simulink model "Cooperative_Quad_09_VelEst_02"  (R2017b)
settings: Solver=ode45  StartTime=0.0  StopTime=120  RelTol=1e-3  EnableMultiTasking=on
InitFcn:
  | Const_Vel_Est_02
values from neighbouring files (symbols this model uses):
  alpha = 1.0e-5    (= 1e-05)    [Cons_AMFC_Quad_New_01.m]    (also in Const_Vel_Est_02.m = 0.1; constant_Rev01_4Agents_10.m = 0.1; constant_Rev01_4Agents_9.m = 0.1)
  alpha_Slid = 0.01    [Cons_AMFC_Quad_New_01.m]    (also in Const_Vel_Est_02.m)
  AN = [     0 1 0 0 ... (first row only)    [Const_Vel_Est_02.m]    (also in constant_Rev01_4Agents_10.m; constant_Rev01_4Agents_9.m)
  B = 1e+0*eye(n)    [Cons_AMFC_Quad_New_01.m]    (also in Const_Vel_Est_02.m = 1e0*eye(n); constant_Rev01_4Agents_10.m = 1e0*eye(n); constant_Rev01_4Agents_9.m = 1e0*eye(n))
  BBT_inv = ((B'*B)^(-1))*B'    [Cons_AMFC_Quad_New_01.m]    (also in Const_Vel_Est_02.m; constant_Rev01_4Agents_10.m; constant_Rev01_4Agents_9.m)
  BN = [     1 0 0 0 ... (first row only)    [Const_Vel_Est_02.m]    (also in constant_Rev01_4Agents_10.m; constant_Rev01_4Agents_9.m)
  epsilon_struct = struct('data',epsilon_InitVal)    [Const_Vel_Est_02.m]    (also in constant_Rev01_4Agents_10.m; constant_Rev01_4Agents_9.m)
  g = 9.81    [Const_Vel_Est_02.m]    (also in Swing2d_01_const.m; constant_Rev01_4Agents_10.m; constant_Rev01_4Agents_9.m)
  gamma_0 = 1e-0*diag([1e-3*ones(3,1);1e-0*ones(3,1)])    [Cons_AMFC_Quad_New_01.m]    (also in Const_Vel_Est_02.m = 1e-1*diag([1e-3*ones(3,1);1e-0*ones(3,1)]); constant_Rev01_4Agents_10.m = 1e+1*diag([1e-3*ones(3,1);1e-0*ones(3,1)]); constant_Rev01_4Agents_9.m = 1e+1*diag([1e-3*ones(6,1);1e-0*ones(6,1)]))
  gamma_1 = 1e+2*diag([1e-3*ones(3,1);1e-0*ones(3,1)])    [Cons_AMFC_Quad_New_01.m]    (also in Const_Vel_Est_02.m; constant_Rev01_4Agents_10.m = 1e+3*diag([1e-3*ones(3,1);1e0*ones(3,1)]); constant_Rev01_4Agents_9.m = 1e+3*diag([1e-3*ones(6,1);1e0*ones(6,1)]))
  H = L + BN    [Const_Vel_Est_02.m]    (also in constant_Rev01_4Agents_10.m; constant_Rev01_4Agents_9.m)
  J = 1.2416e-3 * diag([1 1 2])    [Cons_AMFC_Quad_New_01.m]    (also in Const_Vel_Est_02.m = 1.2416e-3 * diag([1 1 2],0); constant_Rev01_4Agents_10.m = 1.2416e-3 * diag([1 1 2],0); constant_Rev01_4Agents_9.m = 1.2416e-3 * diag([1 1 2],0))
  k1 = 10    [Cons_AMFC_Quad_New_01.m]    (also in Const_Vel_Est_02.m = 1; constant_Rev01_4Agents_10.m = 1; constant_Rev01_4Agents_9.m = 1)
  k1o = 1000    [Cons_AMFC_Quad_New_01.m]    (also in Const_Vel_Est_02.m)
  k2 = 0.1    [Cons_AMFC_Quad_New_01.m]    (also in Const_Vel_Est_02.m; constant_Rev01_4Agents_10.m = 1; constant_Rev01_4Agents_9.m = 1)
  k2o = 100    [Cons_AMFC_Quad_New_01.m]    (also in Const_Vel_Est_02.m)
  Ka = 0.01    [Cons_AMFC_Quad_New_01.m]    (also in Const_Vel_Est_02.m; constant_Rev01_4Agents_10.m; constant_Rev01_4Agents_9.m)
  Kd = 0.01    [Cons_AMFC_Quad_New_01.m]    (also in Const_Vel_Est_02.m; constant_Rev01_4Agents_10.m; constant_Rev01_4Agents_9.m)
  Kf = 1.0e-5    (= 1e-05)    [Cons_AMFC_Quad_New_01.m]    (also in Const_Vel_Est_02.m; constant_Rev01_4Agents_10.m; constant_Rev01_4Agents_9.m)
  Kt = 0.0435 * Kf    (= 4.35e-07)    [Cons_AMFC_Quad_New_01.m]    (also in Const_Vel_Est_02.m = 1e-07; constant_Rev01_4Agents_10.m = 1e-07; constant_Rev01_4Agents_9.m = 1e-07)
  Lq = 0.2    [Const_Vel_Est_02.m]    (also in constant_Rev01_4Agents_10.m; constant_Rev01_4Agents_9.m)
  m = 6    [Cons_AMFC_Quad_New_01.m]    (also in Const_Vel_Est_02.m; Swing2d_01_const.m = 1)
  M = 2.95    [Cons_AMFC_Quad_New_01.m]    (also in Const_Vel_Est_02.m = 2; constant_Rev01_4Agents_10.m = 2; constant_Rev01_4Agents_9.m = 2)
  Mb_P = Mb_val_P*ones(np,1)    [Const_Vel_Est_02.m]
  Mb_V = Mb_val_V*ones(np,1)    [Const_Vel_Est_02.m]
  Mu_P = 10    [Const_Vel_Est_02.m]
  Mu_V = 10    [Const_Vel_Est_02.m]
  n = 6    [Cons_AMFC_Quad_New_01.m]    (also in Const_Vel_Est_02.m; constant_Rev01_4Agents_10.m; constant_Rev01_4Agents_9.m = 12)
  N = 4    [Const_Vel_Est_02.m]    (also in constant_Rev01_4Agents_10.m; constant_Rev01_4Agents_9.m)
  n0 = 3    [Const_Vel_Est_02.m]    (also in constant_Rev01_4Agents_10.m; constant_Rev01_4Agents_9.m)
  np = 2    [Const_Vel_Est_02.m]
  Observer_Gain = 100    [Const_Vel_Est_02.m]    (also in constant_Rev01_4Agents_10.m; constant_Rev01_4Agents_9.m)
  Observer_Gain1 = 100    [Const_Vel_Est_02.m]    (also in constant_Rev01_4Agents_10.m = 10; constant_Rev01_4Agents_9.m = 10)
  Q = 1e-1*eye(n)    [Cons_AMFC_Quad_New_01.m]    (also in Const_Vel_Est_02.m = 1e-2*eye(n); constant_Rev01_4Agents_10.m = 1e-3*eye(n); constant_Rev01_4Agents_9.m = 1e-3*eye(n))
  R = 1e+0*eye(m)    [Cons_AMFC_Quad_New_01.m]    (also in Const_Vel_Est_02.m = 1e-0*eye(n); constant_Rev01_4Agents_10.m = 1e-0*eye(n); constant_Rev01_4Agents_9.m = 1e-0*eye(n))
  rho_0 = 1e-1    (= 0.1)    [Cons_AMFC_Quad_New_01.m]    (also in Const_Vel_Est_02.m; constant_Rev01_4Agents_10.m = 10; constant_Rev01_4Agents_9.m = 10)
  rho_1 = 1e-0    (= 1)    [Cons_AMFC_Quad_New_01.m]    (also in Const_Vel_Est_02.m; constant_Rev01_4Agents_10.m = 0.1; constant_Rev01_4Agents_9.m = 0.1)
  T_struct = struct('data',T_InitVal)    [Const_Vel_Est_02.m]    (also in constant_Rev01_4Agents_10.m; constant_Rev01_4Agents_9.m)
  U_dot0_M = U_dot0_m*ones(n0,1)    [Const_Vel_Est_02.m]    (also in constant_Rev01_4Agents_10.m; constant_Rev01_4Agents_9.m)
  Upsilon_M = Upsilon_m*ones(n0,1)    [Const_Vel_Est_02.m]    (also in constant_Rev01_4Agents_10.m; constant_Rev01_4Agents_9.m)
undefined symbols (not defined in the file or in its folder): sigbuilder_block
(part 3 of 5)

== system Cooperative_Quad_09_VelEst_02/Agent #2/Relative estimations-2/Rel_24/Differentiator1 ==
  x_d : Inport
  Constant : Constant  Value=zeros(3,1)
  Gain : Gain
  Integrator : Integrator
  Integrator1 : Integrator
  Sliding differentiator : MATLAB Function  TreatAsAtomicUnit=on
  Sliding differentiator1 : MATLAB Function  TreatAsAtomicUnit=on
  Sum : Sum  Inputs=|-+
  Dx_d : Outport
  wires:
  Sliding differentiator/1(u) -> Integrator1/1, Dx_d/1
  Gain/1 -> Sum/2
  Integrator1/1 -> Gain/1
  Sum/1 -> Sliding differentiator1/1(e), Sliding differentiator/2(e)
  x_d/1 -> Sum/1
  Integrator/1 -> Sliding differentiator/1(u1)
  Sliding differentiator1/1(Du1) -> Integrator/1

== system Cooperative_Quad_09_VelEst_02/Agent #3/Decenteralized Cooperaive Controller #3/Ali-3/Rotational-3 ==
  x_rd : Inport
  X : Inport  Port=2
  CARE : MATLAB Function  TreatAsAtomicUnit=on
  Differentiator : Subsystem
  Integrator : Integrator  InitialCondition=zeros(n)
  Integrator1 : Integrator  InitialCondition=eye(n)
  Integrator2 : Integrator  InitialCondition=zeros(n,1)
  Integrator3 : Integrator  InitialCondition=zeros(n,1)
  Memory : Memory  InitialCondition=zeros(m,1)
  Sum : Sum  Inputs=|++
  g-Estimator : MATLAB Function  TreatAsAtomicUnit=on
  g-Estimator1 : MATLAB Function  TreatAsAtomicUnit=on
  main : MATLAB Function  TreatAsAtomicUnit=on
  variable change : MATLAB Function  TreatAsAtomicUnit=on
  ur : Outport
  tag scope: A_hat3_R=global, P3_R=global, g_hat3_R=global, u3_R=global
  wires:
  x_rd/1 -> variable change/2(Xd)
  X/1 -> variable change/1(X)
  CARE/1(DP) -> Integrator1/1
  Sum/1 -> main/1(sigma), g-Estimator/1(sigma), g-Estimator1/1(sigma)
  g-Estimator1/1(Da_hat) -> Integrator/1
  variable change/1(x_mod) -> main/7(x), g-Estimator1/2(x)
  Integrator1/1 -> [P3_R], g-Estimator1/3(P), CARE/1(P), g-Estimator/3(P), main/4(P)
  Integrator/1 -> g-Estimator1/4(a_hat), CARE/2(a_hat), [A_hat3_R], main/5(a_hat)
  g-Estimator/1(Dg_hat) -> Integrator2/1
  Differentiator/1(Dx_d) -> main/3(Dy_d)
  main/1(u) -> [u3_R], Memory/1, ur/1
  Integrator3/1 -> main/2(zeta), Sum/1
  variable change/2(xd_mod) -> Differentiator/1(x_d)
  variable change/3(e_mod) -> Sum/2, Integrator3/1
  Memory/1 -> variable change/3(u)
  Integrator2/1 -> g-Estimator/2(g_hat), [g_hat3_R], main/6(g_hat)

== system Cooperative_Quad_09_VelEst_02/Agent #3/Decenteralized Cooperaive Controller #3/Ali-3/Translational-3 ==
  x_td : Inport
  x_t : Inport  Port=2
  A-Estimator : MATLAB Function  TreatAsAtomicUnit=on
  CARE : MATLAB Function  TreatAsAtomicUnit=on
  Differentiator : Subsystem
  Integrator : Integrator  InitialCondition=zeros(n)
  Integrator1 : Integrator  InitialCondition=eye(n)
  Integrator2 : Integrator  InitialCondition=zeros(n,1)
  Integrator3 : Integrator  InitialCondition=zeros(n,1)
  Memory : Memory  InitialCondition=zeros(m,1)
  Sum : Sum  Inputs=|++
  g-Estimator : MATLAB Function  TreatAsAtomicUnit=on
  main : MATLAB Function  TreatAsAtomicUnit=on
  variable change : MATLAB Function  TreatAsAtomicUnit=on
  ut : Outport
  tag scope: A_hat3_T=global, P3_T=global, g_hat3_T=global, u3_T=global
  wires:
  Integrator2/1 -> [g_hat3_T], main/6(g_hat), g-Estimator/2(g_hat)
  Memory/1 -> variable change/3(u)
  variable change/3(e_mod) -> Integrator3/1, Sum/2
  variable change/2(xd_mod) -> Differentiator/1(x_d)
  Integrator3/1 -> Sum/1, main/2(zeta)
  main/1(u) -> ut/1, [u3_T], Memory/1
  Differentiator/1(Dx_d) -> main/3(Dy_d)
  g-Estimator/1(Dg_hat) -> Integrator2/1
  Integrator/1 -> [A_hat3_T], main/5(a_hat), CARE/2(a_hat), A-Estimator/4(a_hat)
  Integrator1/1 -> main/4(P), g-Estimator/3(P), CARE/1(P), [P3_T], A-Estimator/3(P)
  variable change/1(x_mod) -> A-Estimator/2(x), main/7(x)
  A-Estimator/1(Da_hat) -> Integrator/1
  Sum/1 -> A-Estimator/1(sigma), g-Estimator/1(sigma), main/1(sigma)
  CARE/1(DP) -> Integrator1/1
  x_td/1 -> variable change/2(Xd)
  x_t/1 -> variable change/1(X)

== system Cooperative_Quad_09_VelEst_02/Agent #3/Decenteralized Cooperaive Controller #3/Cooperative Observers for X-3/Differentiator2 ==
  Pos_Z : Inport
  Integrator : Integrator
  Integrator1 : Integrator
  Sliding differentiator : MATLAB Function  TreatAsAtomicUnit=on
  Sliding differentiator1 : MATLAB Function  TreatAsAtomicUnit=on
  Sum : Sum  Inputs=|-+
  DPos_Z : Outport
  wires:
  Sliding differentiator/1(u) -> Integrator1/1, DPos_Z/1
  Integrator1/1 -> Sum/2
  Sum/1 -> Sliding differentiator1/1(e), Sliding differentiator/2(e)
  Pos_Z/1 -> Sum/1
  Integrator/1 -> Sliding differentiator/1(u1)
  Sliding differentiator1/1(Du1) -> Integrator/1

== system Cooperative_Quad_09_VelEst_02/Agent #3/Relative estimations-3/Rel_30/Differentiator1 ==
  x_d : Inport
  Constant : Constant  Value=zeros(3,1)
  Gain : Gain
  Integrator : Integrator
  Integrator1 : Integrator
  Sliding differentiator : MATLAB Function  TreatAsAtomicUnit=on
  Sliding differentiator1 : MATLAB Function  TreatAsAtomicUnit=on
  Sum : Sum  Inputs=|-+
  Dx_d : Outport
  wires:
  Sliding differentiator/1(u) -> Integrator1/1, Dx_d/1
  Gain/1 -> Sum/2
  Integrator1/1 -> Gain/1
  Sum/1 -> Sliding differentiator1/1(e), Sliding differentiator/2(e)
  x_d/1 -> Sum/1
  Integrator/1 -> Sliding differentiator/1(u1)
  Sliding differentiator1/1(Du1) -> Integrator/1

== system Cooperative_Quad_09_VelEst_02/Agent #3/Relative estimations-3/Rel_31/Differentiator1 ==
  x_d : Inport
  Constant : Constant  Value=zeros(3,1)
  Gain : Gain
  Integrator : Integrator
  Integrator1 : Integrator
  Sliding differentiator : MATLAB Function  TreatAsAtomicUnit=on
  Sliding differentiator1 : MATLAB Function  TreatAsAtomicUnit=on
  Sum : Sum  Inputs=|-+
  Dx_d : Outport
  wires:
  Sliding differentiator1/1(Du1) -> Integrator/1
  Integrator/1 -> Sliding differentiator/1(u1)
  x_d/1 -> Sum/1
  Sum/1 -> Sliding differentiator/2(e), Sliding differentiator1/1(e)
  Integrator1/1 -> Gain/1
  Gain/1 -> Sum/2
  Sliding differentiator/1(u) -> Dx_d/1, Integrator1/1

== system Cooperative_Quad_09_VelEst_02/Agent #3/Relative estimations-3/Rel_32/Differentiator1 ==
  x_d : Inport
  Constant : Constant  Value=zeros(3,1)
  Gain : Gain
  Integrator : Integrator
  Integrator1 : Integrator
  Sliding differentiator : MATLAB Function  TreatAsAtomicUnit=on
  Sliding differentiator1 : MATLAB Function  TreatAsAtomicUnit=on
  Sum : Sum  Inputs=|-+
  Dx_d : Outport
  wires:
  Sliding differentiator/1(u) -> Integrator1/1, Dx_d/1
  Gain/1 -> Sum/2
  Integrator1/1 -> Gain/1
  Sum/1 -> Sliding differentiator1/1(e), Sliding differentiator/2(e)
  x_d/1 -> Sum/1
  Integrator/1 -> Sliding differentiator/1(u1)
  Sliding differentiator1/1(Du1) -> Integrator/1

== system Cooperative_Quad_09_VelEst_02/Agent #3/Relative estimations-3/Rel_34/Differentiator1 ==
  x_d : Inport
  Constant : Constant  Value=zeros(3,1)
  Gain : Gain
  Integrator : Integrator
  Integrator1 : Integrator
  Sliding differentiator : MATLAB Function  TreatAsAtomicUnit=on
  Sliding differentiator1 : MATLAB Function  TreatAsAtomicUnit=on
  Sum : Sum  Inputs=|-+
  Dx_d : Outport
  wires:
  Sliding differentiator1/1(Du1) -> Integrator/1
  Integrator/1 -> Sliding differentiator/1(u1)
  x_d/1 -> Sum/1
  Sum/1 -> Sliding differentiator/2(e), Sliding differentiator1/1(e)
  Integrator1/1 -> Gain/1
  Gain/1 -> Sum/2
  Sliding differentiator/1(u) -> Dx_d/1, Integrator1/1

== system Cooperative_Quad_09_VelEst_02/Agent #4/Decenteralized Cooperaive Controller #4/Ali-4/Rotational-4 ==
  x_rd : Inport
  X : Inport  Port=2
  CARE : MATLAB Function  TreatAsAtomicUnit=on
  Differentiator : Subsystem
  Integrator : Integrator  InitialCondition=zeros(n)
  Integrator1 : Integrator  InitialCondition=eye(n)
  Integrator2 : Integrator  InitialCondition=zeros(n,1)
  Integrator3 : Integrator  InitialCondition=zeros(n,1)
  Memory : Memory  InitialCondition=zeros(m,1)
  Sum : Sum  Inputs=|++
  g-Estimator : MATLAB Function  TreatAsAtomicUnit=on
  g-Estimator1 : MATLAB Function  TreatAsAtomicUnit=on
  main : MATLAB Function  TreatAsAtomicUnit=on
  variable change : MATLAB Function  TreatAsAtomicUnit=on
  ur : Outport
  tag scope: A_hat4_R=global, P4_R=global, g_hat4_R=global, u4_R=global
  wires:
  Integrator2/1 -> main/6(g_hat), [g_hat4_R], g-Estimator/2(g_hat)
  Memory/1 -> variable change/3(u)
  variable change/3(e_mod) -> Integrator3/1, Sum/2
  variable change/2(xd_mod) -> Differentiator/1(x_d)
  Integrator3/1 -> Sum/1, main/2(zeta)
  main/1(u) -> ur/1, Memory/1, [u4_R]
  Differentiator/1(Dx_d) -> main/3(Dy_d)
  g-Estimator/1(Dg_hat) -> Integrator2/1
  Integrator/1 -> main/5(a_hat), [A_hat4_R], CARE/2(a_hat), g-Estimator1/4(a_hat)
  Integrator1/1 -> main/4(P), g-Estimator/3(P), CARE/1(P), g-Estimator1/3(P), [P4_R]
  variable change/1(x_mod) -> g-Estimator1/2(x), main/7(x)
  g-Estimator1/1(Da_hat) -> Integrator/1
  Sum/1 -> g-Estimator1/1(sigma), g-Estimator/1(sigma), main/1(sigma)
  CARE/1(DP) -> Integrator1/1
  X/1 -> variable change/1(X)
  x_rd/1 -> variable change/2(Xd)

== system Cooperative_Quad_09_VelEst_02/Agent #4/Decenteralized Cooperaive Controller #4/Ali-4/Translational-4 ==
  x_td : Inport
  x_t : Inport  Port=2
  A-Estimator : MATLAB Function  TreatAsAtomicUnit=on
  CARE : MATLAB Function  TreatAsAtomicUnit=on
  Differentiator : Subsystem
  Integrator : Integrator  InitialCondition=zeros(n)
  Integrator1 : Integrator  InitialCondition=eye(n)
  Integrator2 : Integrator  InitialCondition=zeros(n,1)
  Integrator3 : Integrator  InitialCondition=zeros(n,1)
  Memory : Memory  InitialCondition=zeros(m,1)
  Sum : Sum  Inputs=|++
  g-Estimator : MATLAB Function  TreatAsAtomicUnit=on
  main : MATLAB Function  TreatAsAtomicUnit=on
  variable change : MATLAB Function  TreatAsAtomicUnit=on
  ut : Outport
  tag scope: A_hat4_T=global, P4_T=global, g_hat4_T=global, u4_T=global
  wires:
  x_t/1 -> variable change/1(X)
  x_td/1 -> variable change/2(Xd)
  CARE/1(DP) -> Integrator1/1
  Sum/1 -> main/1(sigma), g-Estimator/1(sigma), A-Estimator/1(sigma)
  A-Estimator/1(Da_hat) -> Integrator/1
  variable change/1(x_mod) -> main/7(x), A-Estimator/2(x)
  Integrator1/1 -> A-Estimator/3(P), [P4_T], CARE/1(P), g-Estimator/3(P), main/4(P)
  Integrator/1 -> A-Estimator/4(a_hat), CARE/2(a_hat), main/5(a_hat), [A_hat4_T]
  g-Estimator/1(Dg_hat) -> Integrator2/1
  Differentiator/1(Dx_d) -> main/3(Dy_d)
  main/1(u) -> Memory/1, [u4_T], ut/1
  Integrator3/1 -> main/2(zeta), Sum/1
  variable change/2(xd_mod) -> Differentiator/1(x_d)
  variable change/3(e_mod) -> Sum/2, Integrator3/1
  Memory/1 -> variable change/3(u)
  Integrator2/1 -> g-Estimator/2(g_hat), main/6(g_hat), [g_hat4_T]

== system Cooperative_Quad_09_VelEst_02/Agent #4/Decenteralized Cooperaive Controller #4/Cooperative Observers for X-4/Differentiator2 ==
  Pos_Z : Inport
  Integrator : Integrator
  Integrator1 : Integrator
  Sliding differentiator : MATLAB Function  TreatAsAtomicUnit=on
  Sliding differentiator1 : MATLAB Function  TreatAsAtomicUnit=on
  Sum : Sum  Inputs=|-+
  DPos_Z : Outport
  wires:
  Sliding differentiator1/1(Du1) -> Integrator/1
  Integrator/1 -> Sliding differentiator/1(u1)
  Pos_Z/1 -> Sum/1
  Sum/1 -> Sliding differentiator/2(e), Sliding differentiator1/1(e)
  Integrator1/1 -> Sum/2
  Sliding differentiator/1(u) -> DPos_Z/1, Integrator1/1

== system Cooperative_Quad_09_VelEst_02/Agent #4/Relative estimations-4/Rel_40/Differentiator1 ==
  x_d : Inport
  Constant : Constant  Value=zeros(3,1)
  Gain : Gain
  Integrator : Integrator
  Integrator1 : Integrator
  Sliding differentiator : MATLAB Function  TreatAsAtomicUnit=on
  Sliding differentiator1 : MATLAB Function  TreatAsAtomicUnit=on
  Sum : Sum  Inputs=|-+
  Dx_d : Outport
  wires:
  Sliding differentiator1/1(Du1) -> Integrator/1
  Integrator/1 -> Sliding differentiator/1(u1)
  x_d/1 -> Sum/1
  Sum/1 -> Sliding differentiator/2(e), Sliding differentiator1/1(e)
  Integrator1/1 -> Gain/1
  Gain/1 -> Sum/2
  Sliding differentiator/1(u) -> Dx_d/1, Integrator1/1

== system Cooperative_Quad_09_VelEst_02/Agent #4/Relative estimations-4/Rel_41/Differentiator1 ==
  x_d : Inport
  Constant : Constant  Value=zeros(3,1)
  Gain : Gain
  Integrator : Integrator
  Integrator1 : Integrator
  Sliding differentiator : MATLAB Function  TreatAsAtomicUnit=on
  Sliding differentiator1 : MATLAB Function  TreatAsAtomicUnit=on
  Sum : Sum  Inputs=|-+
  Dx_d : Outport
  wires:
  Sliding differentiator/1(u) -> Integrator1/1, Dx_d/1
  Gain/1 -> Sum/2
  Integrator1/1 -> Gain/1
  Sum/1 -> Sliding differentiator1/1(e), Sliding differentiator/2(e)
  x_d/1 -> Sum/1
  Integrator/1 -> Sliding differentiator/1(u1)
  Sliding differentiator1/1(Du1) -> Integrator/1

== system Cooperative_Quad_09_VelEst_02/Agent #4/Relative estimations-4/Rel_42/Differentiator1 ==
  x_d : Inport
  Constant : Constant  Value=zeros(3,1)
  Gain : Gain
  Integrator : Integrator
  Integrator1 : Integrator
  Sliding differentiator : MATLAB Function  TreatAsAtomicUnit=on
  Sliding differentiator1 : MATLAB Function  TreatAsAtomicUnit=on
  Sum : Sum  Inputs=|-+
  Dx_d : Outport
  wires:
  Sliding differentiator1/1(Du1) -> Integrator/1
  Integrator/1 -> Sliding differentiator/1(u1)
  x_d/1 -> Sum/1
  Sum/1 -> Sliding differentiator/2(e), Sliding differentiator1/1(e)
  Integrator1/1 -> Gain/1
  Gain/1 -> Sum/2
  Sliding differentiator/1(u) -> Dx_d/1, Integrator1/1

== system Cooperative_Quad_09_VelEst_02/Agent #4/Relative estimations-4/Rel_43/Differentiator1 ==
  x_d : Inport
  Constant : Constant  Value=zeros(3,1)
  Gain : Gain
  Integrator : Integrator
  Integrator1 : Integrator
  Sliding differentiator : MATLAB Function  TreatAsAtomicUnit=on
  Sliding differentiator1 : MATLAB Function  TreatAsAtomicUnit=on
  Sum : Sum  Inputs=|-+
  Dx_d : Outport
  wires:
  Sliding differentiator/1(u) -> Integrator1/1, Dx_d/1
  Gain/1 -> Sum/2
  Integrator1/1 -> Gain/1
  Sum/1 -> Sliding differentiator1/1(e), Sliding differentiator/2(e)
  x_d/1 -> Sum/1
  Integrator/1 -> Sliding differentiator/1(u1)
  Sliding differentiator1/1(Du1) -> Integrator/1

== system Cooperative_Quad_09_VelEst_02/Agent #1/Decenteralized Cooperaive Controller #1/Ali-1/Rotational-1/Differentiator ==
  x_d : Inport
  Integrator : Integrator  InitialCondition=zeros(n,1)
  Integrator1 : Integrator  InitialCondition=zeros(n,1)
  Sliding differentiator : MATLAB Function  TreatAsAtomicUnit=on
  Sliding differentiator1 : MATLAB Function  TreatAsAtomicUnit=on
  Sum : Sum  Inputs=|-+
  Dx_d : Outport
  wires:
  Sliding differentiator/1(u) -> Integrator1/1, Dx_d/1
  Sliding differentiator1/1(Du1) -> Integrator/1
  Integrator/1 -> Sliding differentiator/1(u1)
  x_d/1 -> Sum/1
  Sum/1 -> Sliding differentiator/2(e), Sliding differentiator1/1(e)
  Integrator1/1 -> Sum/2

== system Cooperative_Quad_09_VelEst_02/Agent #1/Decenteralized Cooperaive Controller #1/Ali-1/Translational-1/Differentiator ==
  x_d : Inport
  Integrator : Integrator  InitialCondition=zeros(n,1)
  Integrator1 : Integrator  InitialCondition=zeros(n,1)
  Scope : Scope
  Scope1 : Scope
  Sliding differentiator : MATLAB Function  TreatAsAtomicUnit=on
  Sliding differentiator1 : MATLAB Function  TreatAsAtomicUnit=on
  Sum : Sum  Inputs=|-+
  Dx_d : Outport
  wires:
  Integrator1/1 -> Sum/2
  Sum/1 -> Sliding differentiator1/1(e), Sliding differentiator/2(e), Scope1/1
  x_d/1 -> Sum/1
  Integrator/1 -> Sliding differentiator/1(u1)
  Sliding differentiator1/1(Du1) -> Integrator/1
  Sliding differentiator/1(u) -> Dx_d/1, Integrator1/1, Scope/1

== system Cooperative_Quad_09_VelEst_02/Agent #2/Decenteralized Cooperaive Controller #2/Ali-2/Rotational-2/Differentiator ==
  x_d : Inport
  Integrator : Integrator  InitialCondition=zeros(n,1)
  Integrator1 : Integrator  InitialCondition=zeros(n,1)
  Sliding differentiator : MATLAB Function  TreatAsAtomicUnit=on
  Sliding differentiator1 : MATLAB Function  TreatAsAtomicUnit=on
  Sum : Sum  Inputs=|-+
  Dx_d : Outport
  wires:
  Integrator1/1 -> Sum/2
  Sum/1 -> Sliding differentiator1/1(e), Sliding differentiator/2(e)
  x_d/1 -> Sum/1
  Integrator/1 -> Sliding differentiator/1(u1)
  Sliding differentiator1/1(Du1) -> Integrator/1
  Sliding differentiator/1(u) -> Dx_d/1, Integrator1/1

== system Cooperative_Quad_09_VelEst_02/Agent #2/Decenteralized Cooperaive Controller #2/Ali-2/Translational-2/Differentiator ==
  x_d : Inport
  Integrator : Integrator  InitialCondition=zeros(n,1)
  Integrator1 : Integrator  InitialCondition=zeros(n,1)
  Scope : Scope
  Scope1 : Scope
  Sliding differentiator : MATLAB Function  TreatAsAtomicUnit=on
  Sliding differentiator1 : MATLAB Function  TreatAsAtomicUnit=on
  Sum : Sum  Inputs=|-+
  Dx_d : Outport
  wires:
  Sliding differentiator/1(u) -> Scope/1, Integrator1/1, Dx_d/1
  Sliding differentiator1/1(Du1) -> Integrator/1
  Integrator/1 -> Sliding differentiator/1(u1)
  x_d/1 -> Sum/1
  Sum/1 -> Scope1/1, Sliding differentiator/2(e), Sliding differentiator1/1(e)
  Integrator1/1 -> Sum/2

== system Cooperative_Quad_09_VelEst_02/Agent #3/Decenteralized Cooperaive Controller #3/Ali-3/Rotational-3/Differentiator ==
  x_d : Inport
  Integrator : Integrator  InitialCondition=zeros(n,1)
  Integrator1 : Integrator  InitialCondition=zeros(n,1)
  Sliding differentiator : MATLAB Function  TreatAsAtomicUnit=on
  Sliding differentiator1 : MATLAB Function  TreatAsAtomicUnit=on
  Sum : Sum  Inputs=|-+
  Dx_d : Outport
  wires:
  Sliding differentiator/1(u) -> Integrator1/1, Dx_d/1
  Sliding differentiator1/1(Du1) -> Integrator/1
  Integrator/1 -> Sliding differentiator/1(u1)
  x_d/1 -> Sum/1
  Sum/1 -> Sliding differentiator/2(e), Sliding differentiator1/1(e)
  Integrator1/1 -> Sum/2

== system Cooperative_Quad_09_VelEst_02/Agent #3/Decenteralized Cooperaive Controller #3/Ali-3/Translational-3/Differentiator ==
  x_d : Inport
  Integrator : Integrator  InitialCondition=zeros(n,1)
  Integrator1 : Integrator  InitialCondition=zeros(n,1)
  Scope : Scope
  Scope1 : Scope
  Sliding differentiator : MATLAB Function  TreatAsAtomicUnit=on
  Sliding differentiator1 : MATLAB Function  TreatAsAtomicUnit=on
  Sum : Sum  Inputs=|-+
  Dx_d : Outport
  wires:
  Integrator1/1 -> Sum/2
  Sum/1 -> Sliding differentiator1/1(e), Sliding differentiator/2(e), Scope1/1
  x_d/1 -> Sum/1
  Integrator/1 -> Sliding differentiator/1(u1)
  Sliding differentiator1/1(Du1) -> Integrator/1
  Sliding differentiator/1(u) -> Dx_d/1, Integrator1/1, Scope/1

== system Cooperative_Quad_09_VelEst_02/Agent #4/Decenteralized Cooperaive Controller #4/Ali-4/Rotational-4/Differentiator ==
  x_d : Inport
  Integrator : Integrator  InitialCondition=zeros(n,1)
  Integrator1 : Integrator  InitialCondition=zeros(n,1)
  Sliding differentiator : MATLAB Function  TreatAsAtomicUnit=on
  Sliding differentiator1 : MATLAB Function  TreatAsAtomicUnit=on
  Sum : Sum  Inputs=|-+
  Dx_d : Outport
  wires:
  Integrator1/1 -> Sum/2
  Sum/1 -> Sliding differentiator1/1(e), Sliding differentiator/2(e)
  x_d/1 -> Sum/1
  Integrator/1 -> Sliding differentiator/1(u1)
  Sliding differentiator1/1(Du1) -> Integrator/1
  Sliding differentiator/1(u) -> Dx_d/1, Integrator1/1

== system Cooperative_Quad_09_VelEst_02/Agent #4/Decenteralized Cooperaive Controller #4/Ali-4/Translational-4/Differentiator ==
  x_d : Inport
  Integrator : Integrator  InitialCondition=zeros(n,1)
  Integrator1 : Integrator  InitialCondition=zeros(n,1)
  Scope : Scope
  Scope1 : Scope
  Sliding differentiator : MATLAB Function  TreatAsAtomicUnit=on
  Sliding differentiator1 : MATLAB Function  TreatAsAtomicUnit=on
  Sum : Sum  Inputs=|-+
  Dx_d : Outport
  wires:
  Sliding differentiator/1(u) -> Scope/1, Integrator1/1, Dx_d/1
  Sliding differentiator1/1(Du1) -> Integrator/1
  Integrator/1 -> Sliding differentiator/1(u1)
  x_d/1 -> Sum/1
  Sum/1 -> Scope1/1, Sliding differentiator/2(e), Sliding differentiator1/1(e)
  Integrator1/1 -> Sum/2

== matlab function Cooperative_Quad_09_VelEst_02/Agent #1/Decenteralized Cooperaive Controller #1/Ali-1/Controller interpreter-1 ==
  data: u0 output; PHI_d output size=3; u input
function [u0,PHI_d] = fcn(u)

u0 = sqrt((u(4)^2)+(u(5)^2)+(u(6)^2));

psi_d = 0;
phi_d = asin( min(max(((sin(psi_d)*u(4) - cos(psi_d)*u(5)) / (u0+1e-3)),-1),1) );
theta_d = atan( (cos(psi_d)*u(4) + sin(psi_d)*u(5)) / (u(6)+1e-3) );

PHI_d = [phi_d;theta_d;psi_d]; 

end

== matlab function Cooperative_Quad_09_VelEst_02/Agent #1/Decenteralized Cooperaive Controller #1/Computing xd-1  ==
  data: q_i input; T_i input; xd output; Agent_Num input
function xd = fcn(q_i,T_i,Agent_Num)

xd = q_i + T_i(1,:)' + T_i(Agent_Num+1,:)';

end

== matlab function Cooperative_Quad_09_VelEst_02/Agent #2/Decenteralized Cooperaive Controller #2/Ali-2/Controller interpreter-2 ==
  data: u0 output; PHI_d output size=3; u input
function [u0,PHI_d] = fcn(u)

u0 = sqrt((u(4)^2)+(u(5)^2)+(u(6)^2));

psi_d = 0;
phi_d = asin( min(max(((sin(psi_d)*u(4) - cos(psi_d)*u(5)) / (u0+1e-3)),-1),1) );
theta_d = atan( (cos(psi_d)*u(4) + sin(psi_d)*u(5)) / (u(6)+1e-3) );

PHI_d = [phi_d;theta_d;psi_d]; 

end

== matlab function Cooperative_Quad_09_VelEst_02/Agent #2/Decenteralized Cooperaive Controller #2/Ali-2/Controller interpreter1-2 ==
  data: u output; u0t input; ur input; RM_1 parameter
function u = fcn(u0t,ur,RM_1)

y1 = ur(4);
y2 = ur(5);
y3 = ur(6);

Y = [u0t;y1;y2;y3];

u = RM_1*Y;
 
for i=1:4
    u(i) = sqrt(abs(u(i)));
end

end

== matlab function Cooperative_Quad_09_VelEst_02/Agent #2/Decenteralized Cooperaive Controller #2/Ali-2/Rotational-2/CARE ==
  data: P input; a_hat input; B parameter; R parameter; DP output; Q parameter
function DP = fcn(P,a_hat,B,R,Q)

DP = a_hat*P + P*a_hat' - P*B*R*B'*P + 2*Q;

end

== matlab function Cooperative_Quad_09_VelEst_02/Agent #2/Decenteralized Cooperaive Controller #2/Ali-2/Rotational-2/Differentiator/Sliding differentiator ==
  data: u output; u1 input; e input; n parameter; k1 parameter
function u = fcn(u1,e,n,k1)

b=k1;

ABS = zeros(n,1);
for i=1:n
    if e(i)>0
        ABS(i) = e(i);
    else
        ABS(i) = -e(i);
    end
end
SGN = e ./ (ABS + 0.01);

u = u1 - b*(ABS.^0.5).*SGN;

end

== matlab function Cooperative_Quad_09_VelEst_02/Agent #2/Decenteralized Cooperaive Controller #2/Ali-2/Rotational-2/Differentiator/Sliding differentiator1 ==
  data: Du1 output; e input; n parameter; k2 parameter
function Du1 = fcn(e,n,k2)

a=k2;

ABS = zeros(n,1);
for i=1:n
    if e(i)>0
        ABS(i) = e(i);
    else
        ABS(i) = -e(i);
    end
end
SGN = e ./ (ABS + 0.01);

Du1 = - a*SGN;

end

== matlab function Cooperative_Quad_09_VelEst_02/Agent #2/Decenteralized Cooperaive Controller #2/Ali-2/Rotational-2/g-Estimator ==
  data: sigma input; g_hat input; P input; rho_1 parameter; gamma_1 parameter; Dg_hat output
function Dg_hat = fcn(sigma,g_hat,P,rho_1,gamma_1)

Dg_hat = - gamma_1 * P * sigma - rho_1 * gamma_1 * g_hat;

end

== matlab function Cooperative_Quad_09_VelEst_02/Agent #2/Decenteralized Cooperaive Controller #2/Ali-2/Rotational-2/g-Estimator1 ==
  data: sigma input; x input; P input; rho_0 parameter; gamma_0 parameter; Da_hat output; a_hat input
function Da_hat = fcn(sigma,x,P,rho_0,gamma_0,a_hat)

DVa_hat = - gamma_0 * P * diag(sigma) * (x - sigma) - rho_0 * gamma_0 * diag(a_hat);

Da_hat = diag(DVa_hat);

end

== matlab function Cooperative_Quad_09_VelEst_02/Agent #2/Decenteralized Cooperaive Controller #2/Ali-2/Rotational-2/main ==
  data: sigma input; zeta input; u output; Dy_d input; R parameter; P input; a_hat input; B parameter; g_hat input; x input; Q parameter; BBT_inv parameter; n parameter
function u = fcn(sigma,zeta,Dy_d,R,P,a_hat,B,g_hat,x,Q,BBT_inv,n)

u1 = (1/2) * R * B' * P * sigma;
u2 = BBT_inv * (Dy_d - a_hat*x + (eye(n) + 2*(((P)^(-1)*Q)) + a_hat)*sigma - g_hat - zeta) - (3/4) * R * B' * P * sigma;

u = u1 + u2;

end

== matlab function Cooperative_Quad_09_VelEst_02/Agent #1/Decenteralized Cooperaive Controller #1/Cooperative Observers for Xd-1/Observer T#1 ==
  data: T_struct parameter; T input; DT_i output; epsilon input; epsilon_struct parameter; H parameter; BN parameter; AN parameter; T_i input; chi input; Upsilon_M parameter; epsilon_i output; N parameter; n0 parameter; Agent_Num input; Observer_Gain1 parameter; alpha parameter
function [DT_i,epsilon_i] = fcn(T_struct,T,epsilon,epsilon_struct,H,BN,AN,T_i,chi,Upsilon_M,N,n0,...
    Agent_Num,Observer_Gain1,alpha)

T_struct(1).data = T.t1;
T_struct(2).data = T.t2;
T_struct(3).data = T.t3;
T_struct(4).data = T.t4;

epsilon_struct(1).data = epsilon.eps1;
epsilon_struct(2).data = epsilon.eps2;
epsilon_struct(3).data = epsilon.eps3;
epsilon_struct(4).data = epsilon.eps4;

epsilon_i = + BN(Agent_Num,Agent_Num)*(T_i - chi);
Sum2 = zeros(N+1,n0);
for i=1:N
    epsilon_i = epsilon_i + ( AN(Agent_Num,i) * (T_i - T_struct(i).data) );  
    Sum2 = Sum2 + ( H(i,Agent_Num) * epsilon_struct(i).data );
end

Sum21 = abs(Sum2) + alpha;
SGN2 = Sum2./Sum21;

DT_i = -Observer_Gain1*epsilon_i - SGN2*diag(Upsilon_M);

end

== matlab function Cooperative_Quad_09_VelEst_02/Agent #1/Decenteralized Cooperaive Controller #1/Cooperative Observers for Xd-1/Observer q#1 ==
  data: q input; Dq_i output; tau input; H parameter; BN parameter; AN parameter; q_i input; u0 input; U_dot0_M parameter; tau_i output; N parameter; Agent_Num input; Observer_Gain parameter; n0 parameter; alpha parameter
function [Dq_i,tau_i] = fcn(q,tau,H,BN,AN,q_i,u0,U_dot0_M,N,Agent_Num,Observer_Gain,n0,alpha)

tau_i = + BN(Agent_Num,Agent_Num)*(q_i - u0);
Sum2 = zeros(n0,1);
for i=1:N
    tau_i = tau_i + ( AN(Agent_Num,i) * (q_i - q(((i-1)*n0+1):n0*i)) );  
    Sum2 = Sum2 + ( H(i,Agent_Num) * tau(((i-1)*n0+1):n0*i) );
end

Sum21 = abs(Sum2) + alpha;
SGN2 = Sum2./Sum21;

Dq_i = -Observer_Gain*tau_i - diag(SGN2)*U_dot0_M;

end

== matlab function Cooperative_Quad_09_VelEst_02/Agent #2/Decenteralized Cooperaive Controller #2/Ali-2/Rotational-2/variable change ==
  data: X input; Xd input; x_mod output; u input; xd_mod output; e_mod output
function [x_mod,xd_mod,e_mod] = fcn(X,Xd,u)

x_mod = [X(4:6);X(10:12)];

xd_mod = [Xd;u(1:3)];

e_mod = xd_mod - x_mod;


end

== matlab function Cooperative_Quad_09_VelEst_02/Agent #1/Plant #1/MATLAB Function ==
  data: X input; u1 input; u2 input; u3 input; u4 input; t input; DX output; Kf parameter; Kt parameter; Kd parameter; Ka parameter; M parameter; J parameter; Lq parameter; g parameter; Pos_XY output; Pos_Z output; Vel_XY output; Acc_XY output
function [DX,Pos_XY,Pos_Z,Vel_XY,Acc_XY] = fcn(X,u1,u2,u3,u4,t,Kf,Kt,Kd,Ka,M,J,Lq,g)

F1 = Kf * u1^2;
F2 = Kf * u2^2;
F3 = Kf * u3^2;
F4 = Kf * u4^2;
 
FT = F1 + F2 + F3 + F4;

T1 = Kt * u1^2;
T2 = Kt * u2^2;
T3 = Kt * u3^2;
T4 = Kt * u4^2;

phi = X(4);
theta = X(5);
psi = X(6);

Rq = [cos(psi)*cos(theta) -sin(psi)*cos(phi)+cos(psi)*sin(theta)*sin(phi) sin(psi)*sin(phi)+cos(psi)*sin(theta)*cos(phi);
    sin(psi)*cos(theta) cos(psi)*cos(phi)+sin(psi)*sin(theta)*sin(phi) -cos(psi)*sin(phi)+sin(psi)*sin(theta)*cos(phi);
    -sin(theta) cos(theta)*sin(phi) cos(theta)*cos(phi)]; 

R_omega = [1 0 -sin(theta);
    0 cos(phi) cos(theta)*sin(phi);
    0 -sin(phi) cos(theta)*cos(phi)];

EXT_PRD = External_Product3(X(10:12),(J*X(10:12)));

DP = X(7:9);
DPHI = R_omega^(-1) * X(10:12); 
Dv = (1/M)*(Rq*[0;0;FT] - Kd*X(7:9) - M*[0;0;g]) + Rq*(1*sin(1*t))*[0;0;1];
Dw = (J^(-1))*([Lq*(F3-F1);Lq*(F4-F2);(T1-T2+T3-T4)] - Ka*X(10:12) - EXT_PRD) + (1*sin(1*t));

DX = [DP;DPHI;Dv;Dw];

Pos_XY = X(1:2);
Pos_Z = X(3);
Vel_XY = X(7:8);
Acc_XY = DX(7:8);

end

== matlab function Cooperative_Quad_09_VelEst_02/Agent #2/Decenteralized Cooperaive Controller #2/Ali-2/Translational-2/A-Estimator ==
  data: sigma input; x input; P input; rho_0 parameter; gamma_0 parameter; Da_hat output; a_hat input
function Da_hat = fcn(sigma,x,P,rho_0,gamma_0,a_hat)

DVa_hat = - gamma_0 * P * diag(sigma) * (x - sigma) - rho_0 * gamma_0 * diag(a_hat);

Da_hat = diag(DVa_hat);

end

== matlab function Cooperative_Quad_09_VelEst_02/Agent #2/Decenteralized Cooperaive Controller #2/Ali-2/Translational-2/CARE ==
  data: P input; a_hat input; B parameter; R parameter; DP output; Q parameter
function DP = fcn(P,a_hat,B,R,Q)

DP = a_hat*P + P*a_hat' - P*B*R*B'*P + 2*Q;

end

== matlab function Cooperative_Quad_09_VelEst_02/Agent #2/Decenteralized Cooperaive Controller #2/Ali-2/Translational-2/Differentiator/Sliding differentiator ==
  data: u output; u1 input; e input; n parameter; k1 parameter
function u = fcn(u1,e,n,k1)

b=k1;

ABS = zeros(n,1);
for i=1:n
    if e(i)>0
        ABS(i) = e(i);
    else
        ABS(i) = -e(i);
    end
end
SGN = e ./ (ABS + 0.01);

u = u1 - b*(ABS.^0.5).*SGN;

end

== matlab function Cooperative_Quad_09_VelEst_02/Agent #2/Decenteralized Cooperaive Controller #2/Ali-2/Translational-2/Differentiator/Sliding differentiator1 ==
  data: Du1 output; e input; n parameter; k2 parameter
function Du1 = fcn(e,n,k2)

a=k2;

ABS = zeros(n,1);
for i=1:n
    if e(i)>0
        ABS(i) = e(i);
    else
        ABS(i) = -e(i);
    end
end
SGN = e ./ (ABS + 0.01);

Du1 = - a*SGN;

end

== matlab function Cooperative_Quad_09_VelEst_02/Agent #2/Decenteralized Cooperaive Controller #2/Ali-2/Translational-2/g-Estimator ==
  data: sigma input; g_hat input; P input; rho_1 parameter; gamma_1 parameter; Dg_hat output
function Dg_hat = fcn(sigma,g_hat,P,rho_1,gamma_1)

Dg_hat = - gamma_1 * P * sigma - rho_1 * gamma_1 * g_hat;

end

== matlab function Cooperative_Quad_09_VelEst_02/Agent #2/Decenteralized Cooperaive Controller #2/Ali-2/Translational-2/main ==
  data: sigma input; zeta input; u output; Dy_d input; R parameter; P input; a_hat input; B parameter; g_hat input; x input; Q parameter; BBT_inv parameter; n parameter
function u = fcn(sigma,zeta,Dy_d,R,P,a_hat,B,g_hat,x,Q,BBT_inv,n)

u1 = (1/2) * R * B' * P * sigma;
u2 = BBT_inv * (Dy_d - a_hat*x + (eye(n) + 2*(((P)^(-1)*Q)) + a_hat)*sigma - g_hat - zeta) - (3/4) * R * B' * P * sigma;

u = u1 + u2;

end

== matlab function Cooperative_Quad_09_VelEst_02/Agent #2/Decenteralized Cooperaive Controller #2/Ali-2/Translational-2/variable change ==
  data: X input; Xd input; x_mod output; u input; xd_mod output; e_mod output
function [x_mod,xd_mod,e_mod] = fcn(X,Xd,u)

x_mod = [X(1:3);X(7:9)];

xd_mod = [Xd;u(1:3)];

e_mod = xd_mod - x_mod;


end

== matlab function Cooperative_Quad_09_VelEst_02/Agent #2/Decenteralized Cooperaive Controller #2/Computing xd-2  ==
  data: q_i input; T_i input; xd output; Agent_Num input
function xd = fcn(q_i,T_i,Agent_Num)

xd = q_i + T_i(1,:)' + T_i(Agent_Num+1,:)';

end

== matlab function Cooperative_Quad_09_VelEst_02/Agent #2/Decenteralized Cooperaive Controller #2/Cooperative Observers for X-2/Differentiator2/Sliding differentiator ==
  data: u output; u1 input; e input; k1o parameter; alpha_Slid parameter
function u = fcn(u1,e,k1o,alpha_Slid)

b=k1o;

ABS = abs(e);
SGN = e ./ (ABS + alpha_Slid);
u = u1 - b*((ABS.^0.5).*SGN); 

end

== matlab function Cooperative_Quad_09_VelEst_02/Agent #2/Decenteralized Cooperaive Controller #2/Cooperative Observers for X-2/Differentiator2/Sliding differentiator1 ==
  data: Du1 output; e input; k2o parameter; alpha_Slid parameter
function Du1 = fcn(e,k2o,alpha_Slid)

a=k2o;

ABS = abs(e);
SGN = e ./ (ABS + alpha_Slid);
Du1 = - a*SGN;

end

== matlab function Cooperative_Quad_09_VelEst_02/Agent #2/Decenteralized Cooperaive Controller #2/Cooperative Observers for X-2/MATLAB Function ==
  data: X_inp input; X_est output; P_est_XY input; Pos_local_Z input; V_est_XY input; V_local_Z input
function X_est = fcn(X_inp,P_est_XY,Pos_local_Z,V_est_XY,V_local_Z)

X_est = [P_est_XY;Pos_local_Z;X_inp(4:6);V_est_XY;V_local_Z;X_inp(10:12)];

end

== matlab function Cooperative_Quad_09_VelEst_02/Agent #2/Decenteralized Cooperaive Controller #2/Cooperative Observers for X-2/Pos observer-2 ==
  data: P_hat input; tau input; P0 input; P_rel_local input; P_rel0_local input; AN parameter; BN parameter; H parameter; DP_hat_local output; np parameter; N parameter; Num input; Mu_P parameter; Mb_P parameter; tau_i output; alpha parameter
function [DP_hat_local,tau_i] = fcn(P_hat,tau,P0,P_rel_local,P_rel0_local,AN,BN,H,np,N,Num,Mu_P,Mb_P,alpha)

P_hat_in = zeros(np,N);
P_rel_local_in = zeros(np,N);
tau_in = zeros(np,N);
for i=1:N
    P_hat_in(:,i) = P_hat((i-1)*np+1:(i*np),1); 
    P_rel_local_in(:,i) = P_rel_local((i-1)*np+1:(i*np),1); 
    tau_in(:,i) = tau((i-1)*np+1:(i*np),1);
end

e = BN(Num,Num)*(P_hat_in(:,Num) - (P0 + P_rel0_local));
Vec = zeros(np,1);
for i=1:N
    e = e + ( AN(Num,i)*(P_hat_in(:,Num) - (P_hat_in(:,i) + P_rel_local_in(:,i))) ); 
    Vec = Vec + ( H(Num,i)*tau_in(:,i) );    
end

SGN_vec = Vec./(abs(Vec)+alpha);
SGN = diag(SGN_vec);    

DP_hat_local = - ( Mu_P*e ) - ( SGN*Mb_P );
tau_i = e;

end

== matlab function Cooperative_Quad_09_VelEst_02/Agent #2/Decenteralized Cooperaive Controller #2/Cooperative Observers for X-2/Vel observer-2 ==
  data: P_hat input; tau input; P0 input; P_rel_local input; P_rel0_local input; AN parameter; BN parameter; H parameter; DP_hat_local output; np parameter; N parameter; Num input; Mu_V parameter; Mb_V parameter; tau_i output; alpha parameter
function [DP_hat_local,tau_i] = fcn(P_hat,tau,P0,P_rel_local,P_rel0_local,AN,BN,H,np,N,Num,Mu_V,Mb_V,alpha)

P_hat_in = zeros(np,N);
P_rel_local_in = zeros(np,N);
tau_in = zeros(np,N);
for i=1:N
    P_hat_in(:,i) = P_hat((i-1)*np+1:(i*np),1); 
    P_rel_local_in(:,i) = P_rel_local((i-1)*np+1:(i*np),1); 
    tau_in(:,i) = tau((i-1)*np+1:(i*np),1);
end

e = BN(Num,Num)*(P_hat_in(:,Num) - (P0 + P_rel0_local));
Vec = zeros(np,1);
for i=1:N
    e = e + ( AN(Num,i)*(P_hat_in(:,Num) - (P_hat_in(:,i) + P_rel_local_in(:,i))) ); 
    Vec = Vec + ( H(Num,i)*tau_in(:,i) );    
end

SGN_vec = Vec./(abs(Vec)+alpha);
SGN = diag(SGN_vec);    

DP_hat_local = - ( Mu_V*e ) - ( SGN*Mb_V );
tau_i = e;

end

== matlab function Cooperative_Quad_09_VelEst_02/Agent #2/Decenteralized Cooperaive Controller #2/Cooperative Observers for Xd-2/Observer T#2 ==
  data: T_struct parameter; T input; DT_i output; epsilon input; epsilon_struct parameter; H parameter; BN parameter; AN parameter; T_i input; chi input; Upsilon_M parameter; epsilon_i output; N parameter; n0 parameter; Agent_Num input; Observer_Gain1 parameter; alpha parameter
function [DT_i,epsilon_i] = fcn(T_struct,T,epsilon,epsilon_struct,H,BN,AN,T_i,chi,Upsilon_M,N,n0,...
    Agent_Num,Observer_Gain1,alpha)

T_struct(1).data = T.t1;
T_struct(2).data = T.t2;
T_struct(3).data = T.t3;
T_struct(4).data = T.t4;

epsilon_struct(1).data = epsilon.eps1;
epsilon_struct(2).data = epsilon.eps2;
epsilon_struct(3).data = epsilon.eps3;
epsilon_struct(4).data = epsilon.eps4;

epsilon_i = + BN(Agent_Num,Agent_Num)*(T_i - chi);
Sum2 = zeros(N+1,n0);
for i=1:N
    epsilon_i = epsilon_i + ( AN(Agent_Num,i) * (T_i - T_struct(i).data) );  
    Sum2 = Sum2 + ( H(i,Agent_Num) * epsilon_struct(i).data );
end

Sum21 = abs(Sum2) + alpha;
SGN2 = Sum2./Sum21;

DT_i = -Observer_Gain1*epsilon_i - SGN2*diag(Upsilon_M);

end

== matlab function Cooperative_Quad_09_VelEst_02/Agent #2/Decenteralized Cooperaive Controller #2/Cooperative Observers for Xd-2/Observer q#2 ==
  data: q input; Dq_i output; tau input; H parameter; BN parameter; AN parameter; q_i input; u0 input; U_dot0_M parameter; tau_i output; N parameter; Agent_Num input; Observer_Gain parameter; n0 parameter; alpha parameter
function [Dq_i,tau_i] = fcn(q,tau,H,BN,AN,q_i,u0,U_dot0_M,N,Agent_Num,Observer_Gain,n0,alpha)

tau_i = + BN(Agent_Num,Agent_Num)*(q_i - u0);
Sum2 = zeros(n0,1);
for i=1:N
    tau_i = tau_i + ( AN(Agent_Num,i) * (q_i - q(((i-1)*n0+1):n0*i)) );  
    Sum2 = Sum2 + ( H(i,Agent_Num) * tau(((i-1)*n0+1):n0*i) );
end

Sum21 = abs(Sum2) + alpha;
SGN2 = Sum2./Sum21;

Dq_i = -Observer_Gain*tau_i - diag(SGN2)*U_dot0_M;

end

== matlab function Cooperative_Quad_09_VelEst_02/Agent #1/Relative estimations-1/Rel_13/Differentiator1/Sliding differentiator ==
  data: u output; u1 input; e input; k1o parameter; alpha_Slid parameter
function u = fcn(u1,e,k1o,alpha_Slid)

b=k1o;

ABS = abs(e);
SGN = e ./ (ABS + alpha_Slid);
u = u1 - b*((ABS.^0.5).*SGN); 

end

== matlab function Cooperative_Quad_09_VelEst_02/Agent #1/Relative estimations-1/Rel_13/Differentiator1/Sliding differentiator1 ==
  data: Du1 output; e input; k2o parameter; alpha_Slid parameter
function Du1 = fcn(e,k2o,alpha_Slid)

a=k2o;

ABS = abs(e);
SGN = e ./ (ABS + alpha_Slid);
Du1 = - a*SGN;

end

== matlab function Cooperative_Quad_09_VelEst_02/Agent #2/Plant #2/MATLAB Function ==
  data: X input; u1 input; u2 input; u3 input; u4 input; t input; DX output; Kf parameter; Kt parameter; Kd parameter; Ka parameter; M parameter; J parameter; Lq parameter; g parameter; Pos_XY output; Pos_Z output; Vel_XY output; Acc_XY output
function [DX,Pos_XY,Pos_Z,Vel_XY,Acc_XY] = fcn(X,u1,u2,u3,u4,t,Kf,Kt,Kd,Ka,M,J,Lq,g)

F1 = Kf * u1^2;
F2 = Kf * u2^2;
F3 = Kf * u3^2;
F4 = Kf * u4^2;
 
FT = F1 + F2 + F3 + F4;

T1 = Kt * u1^2;
T2 = Kt * u2^2;
T3 = Kt * u3^2;
T4 = Kt * u4^2;

phi = X(4);
theta = X(5);
psi = X(6);

Rq = [cos(psi)*cos(theta) -sin(psi)*cos(phi)+cos(psi)*sin(theta)*sin(phi) sin(psi)*sin(phi)+cos(psi)*sin(theta)*cos(phi);
    sin(psi)*cos(theta) cos(psi)*cos(phi)+sin(psi)*sin(theta)*sin(phi) -cos(psi)*sin(phi)+sin(psi)*sin(theta)*cos(phi);
    -sin(theta) cos(theta)*sin(phi) cos(theta)*cos(phi)]; 

R_omega = [1 0 -sin(theta);
    0 cos(phi) cos(theta)*sin(phi);
    0 -sin(phi) cos(theta)*cos(phi)];

EXT_PRD = External_Product3(X(10:12),(J*X(10:12)));

DP = X(7:9);
DPHI = R_omega^(-1) * X(10:12); 
Dv = (1/M)*(Rq*[0;0;FT] - Kd*X(7:9) - M*[0;0;g]) + Rq*(1*sin(1*t))*[0;0;1];
Dw = (J^(-1))*([Lq*(F3-F1);Lq*(F4-F2);(T1-T2+T3-T4)] - Ka*X(10:12) - EXT_PRD) + (1*sin(1*t));

DX = [DP;DPHI;Dv;Dw];

Pos_XY = X(1:2);
Pos_Z = X(3);
Vel_XY = X(7:8);
Acc_XY = DX(7:8);

end

== matlab function Cooperative_Quad_09_VelEst_02/Agent #2/Relative estimations-2/Rel_20/Differentiator1/Sliding differentiator ==
  data: u output; u1 input; e input; k1o parameter; alpha_Slid parameter
function u = fcn(u1,e,k1o,alpha_Slid)

b=k1o;

ABS = abs(e);
SGN = e ./ (ABS + alpha_Slid);
u = u1 - b*((ABS.^0.5).*SGN); 

end

== matlab function Cooperative_Quad_09_VelEst_02/Agent #2/Relative estimations-2/Rel_20/Differentiator1/Sliding differentiator1 ==
  data: Du1 output; e input; k2o parameter; alpha_Slid parameter
function Du1 = fcn(e,k2o,alpha_Slid)

a=k2o;

ABS = abs(e);
SGN = e ./ (ABS + alpha_Slid);
Du1 = - a*SGN;

end

== matlab function Cooperative_Quad_09_VelEst_02/Agent #2/Relative estimations-2/Rel_20/Relative estimation1 ==
  data: V_rel input; dp input; DP_est output; P_est input; alpha_P parameter
function DP_est = fcn(V_rel,dp,P_est,alpha_P)

ep = (dp^2) - (P_est'*P_est);
gp = P_est'*V_rel;

DP_est = (1 + alpha_P * sign(ep*gp)) * V_rel;

end

== matlab function Cooperative_Quad_09_VelEst_02/Agent #2/Relative estimations-2/Rel_20/Relative estimation2 ==
  data: A_rel input; dv input; DV_est output size=2; V_est input size=2; alpha_V parameter
function DV_est = fcn(A_rel,dv,V_est,alpha_V)

ev = (dv^2) - (V_est'*V_est);
gv = V_est'*A_rel;

DV_est = (1 + alpha_V * sign(ev*gv)) * A_rel;

end

== matlab function Cooperative_Quad_09_VelEst_02/Agent #2/Relative estimations-2/Rel_20/Relative measurements1 ==
  data: P_other input; d output; P_local input
function d = fcn(P_other,P_local)

P2 = P_local;
P1 = P_other;

d = sqrt( (P2(1) - P1(1))^2 + (P2(2) - P1(2))^2 );

end

== matlab function Cooperative_Quad_09_VelEst_02/Agent #2/Relative estimations-2/Rel_21/Differentiator1/Sliding differentiator ==
  data: u output; u1 input; e input; k1o parameter; alpha_Slid parameter
function u = fcn(u1,e,k1o,alpha_Slid)

b=k1o;

ABS = abs(e);
SGN = e ./ (ABS + alpha_Slid);
u = u1 - b*((ABS.^0.5).*SGN); 

end

== matlab function Cooperative_Quad_09_VelEst_02/Agent #2/Relative estimations-2/Rel_21/Differentiator1/Sliding differentiator1 ==
  data: Du1 output; e input; k2o parameter; alpha_Slid parameter
function Du1 = fcn(e,k2o,alpha_Slid)

a=k2o;

ABS = abs(e);
SGN = e ./ (ABS + alpha_Slid);
Du1 = - a*SGN;

end

== matlab function Cooperative_Quad_09_VelEst_02/Agent #2/Relative estimations-2/Rel_21/Relative estimation2 ==
  data: V_rel input; dp input; DP_est output; P_est input; alpha_P parameter
function DP_est = fcn(V_rel,dp,P_est,alpha_P)

ep = (dp^2) - (P_est'*P_est);
gp = P_est'*V_rel;

DP_est = (1 + alpha_P * sign(ep*gp)) * V_rel;

end

== matlab function Cooperative_Quad_09_VelEst_02/Agent #2/Relative estimations-2/Rel_21/Relative estimation1-2 ==
  data: A_rel input; dv input; DV_est output size=2; V_est input size=2; alpha_V parameter
function DV_est = fcn(A_rel,dv,V_est,alpha_V)

ev = (dv^2) - (V_est'*V_est);
gv = V_est'*A_rel;

DV_est = (1 + alpha_V * sign(ev*gv)) * A_rel;

end

== matlab function Cooperative_Quad_09_VelEst_02/Agent #2/Relative estimations-2/Rel_21/Relative measurements2 ==
  data: P_other input; d output; P_local input
function d = fcn(P_other,P_local)

P2 = P_local;
P1 = P_other;

d = sqrt( (P2(1) - P1(1))^2 + (P2(2) - P1(2))^2 );

end

== matlab function Cooperative_Quad_09_VelEst_02/Agent #2/Relative estimations-2/Rel_23/Differentiator1/Sliding differentiator ==
  data: u output; u1 input; e input; k1o parameter; alpha_Slid parameter
function u = fcn(u1,e,k1o,alpha_Slid)

b=k1o;

ABS = abs(e);
SGN = e ./ (ABS + alpha_Slid);
u = u1 - b*((ABS.^0.5).*SGN); 

end

== matlab function Cooperative_Quad_09_VelEst_02/Data Bus /Reference Trajectory/formation ==
  data: r_form_x input; chi output; r_form_y input; r_form_z input
function chi = fcn(r_form_x,r_form_y,r_form_z)

Delta_form = [...
    +r_form_x +r_form_y +r_form_z;
    -r_form_x +r_form_y -r_form_z;
    -r_form_x -r_form_y +2*r_form_z;
    +r_form_x -r_form_y -2*r_form_z];

chi = [0 0 0;
    Delta_form];

end

== matlab function Cooperative_Quad_09_VelEst_02/Agent #1/Decenteralized Cooperaive Controller #1/Ali-1/Controller interpreter1-1 ==
  data: u output; u0t input; ur input; RM_1 parameter
function u = fcn(u0t,ur,RM_1)

y1 = ur(4);
y2 = ur(5);
y3 = ur(6);

Y = [u0t;y1;y2;y3];

u = RM_1*Y;
 
for i=1:4
    u(i) = sqrt(abs(u(i)));
end

end

== matlab function Cooperative_Quad_09_VelEst_02/Agent #1/Decenteralized Cooperaive Controller #1/Ali-1/Rotational-1/CARE ==
  data: P input; a_hat input; B parameter; R parameter; DP output; Q parameter
function DP = fcn(P,a_hat,B,R,Q)

DP = a_hat*P + P*a_hat' - P*B*R*B'*P + 2*Q;

end

== matlab function Cooperative_Quad_09_VelEst_02/Agent #1/Decenteralized Cooperaive Controller #1/Ali-1/Rotational-1/Differentiator/Sliding differentiator ==
  data: u output; u1 input; e input; n parameter; k1 parameter
function u = fcn(u1,e,n,k1)

b=k1;

ABS = zeros(n,1);
for i=1:n
    if e(i)>0
        ABS(i) = e(i);
    else
        ABS(i) = -e(i);
    end
end
SGN = e ./ (ABS + 0.01);

u = u1 - b*(ABS.^0.5).*SGN;

end

== matlab function Cooperative_Quad_09_VelEst_02/Agent #1/Decenteralized Cooperaive Controller #1/Ali-1/Rotational-1/Differentiator/Sliding differentiator1 ==
  data: Du1 output; e input; n parameter; k2 parameter
function Du1 = fcn(e,n,k2)

a=k2;

ABS = zeros(n,1);
for i=1:n
    if e(i)>0
        ABS(i) = e(i);
    else
        ABS(i) = -e(i);
    end
end
SGN = e ./ (ABS + 0.01);

Du1 = - a*SGN;

end

== matlab function Cooperative_Quad_09_VelEst_02/Agent #1/Decenteralized Cooperaive Controller #1/Ali-1/Rotational-1/g-Estimator ==
  data: sigma input; g_hat input; P input; rho_1 parameter; gamma_1 parameter; Dg_hat output
function Dg_hat = fcn(sigma,g_hat,P,rho_1,gamma_1)

Dg_hat = - gamma_1 * P * sigma - rho_1 * gamma_1 * g_hat;

end

== matlab function Cooperative_Quad_09_VelEst_02/Agent #1/Decenteralized Cooperaive Controller #1/Ali-1/Rotational-1/g-Estimator1 ==
  data: sigma input; x input; P input; rho_0 parameter; gamma_0 parameter; Da_hat output; a_hat input
function Da_hat = fcn(sigma,x,P,rho_0,gamma_0,a_hat)

DVa_hat = - gamma_0 * P * diag(sigma) * (x - sigma) - rho_0 * gamma_0 * diag(a_hat);

Da_hat = diag(DVa_hat);

end

== matlab function Cooperative_Quad_09_VelEst_02/Agent #1/Decenteralized Cooperaive Controller #1/Ali-1/Rotational-1/main ==
  data: sigma input; zeta input; u output; Dy_d input; R parameter; P input; a_hat input; B parameter; g_hat input; x input; Q parameter; BBT_inv parameter; n parameter
function u = fcn(sigma,zeta,Dy_d,R,P,a_hat,B,g_hat,x,Q,BBT_inv,n)

u1 = (1/2) * R * B' * P * sigma;
u2 = BBT_inv * (Dy_d - a_hat*x + (eye(n) + 2*(((P)^(-1)*Q)) + a_hat)*sigma - g_hat - zeta) - (3/4) * R * B' * P * sigma;

u = u1 + u2;

end
